simulink model "SIM_NARENDRA_4_METODO_DIFERENCIAL"  (R2012a)
settings: Solver=ode3  StartTime=0.0  StopTime=2.5  FixedStep=1e-4  RelTol=1e-3
libraries: simulink x1
settings Model: Creator=user  LastModifiedBy=user
settings DataIOCC: LimitDataPoints=on  SaveFormat=Array  ReturnWorkspaceOutputs=off
settings OptimizationCC: LifeSpan=inf  SimCompilerOptimization=Off
settings DebuggingCC: FcnCallInpInsideContextMsg=Enable All  SFUnexpectedBacktrackingDiag=warning  SFNoUnconditionalDefaultTransitionDiag=warning
settings HardwareCC: ProdBitPerPointer=32  ProdLargestAtomicFloat=None  ProdIntDivRoundTo=Undefined  ProdEndianess=Unspecified  ProdWordSize=32  ProdHWDeviceType=32-bit Generic
settings ModelReferenceCC: PropagateSignalLabelsOutOfModel=off
settings SFSimCC: SimUseLocalCustomCode=off
settings RTWCC: RTWUseLocalCustomCode=off  RTWCompilerOptimization=Off
settings GRTTargetCC: CodeReplacementLibrary=C89/C90 (ANSI)  GeneratePreprocessorConditionals=Disable all  CPPClassGenCompliant=off

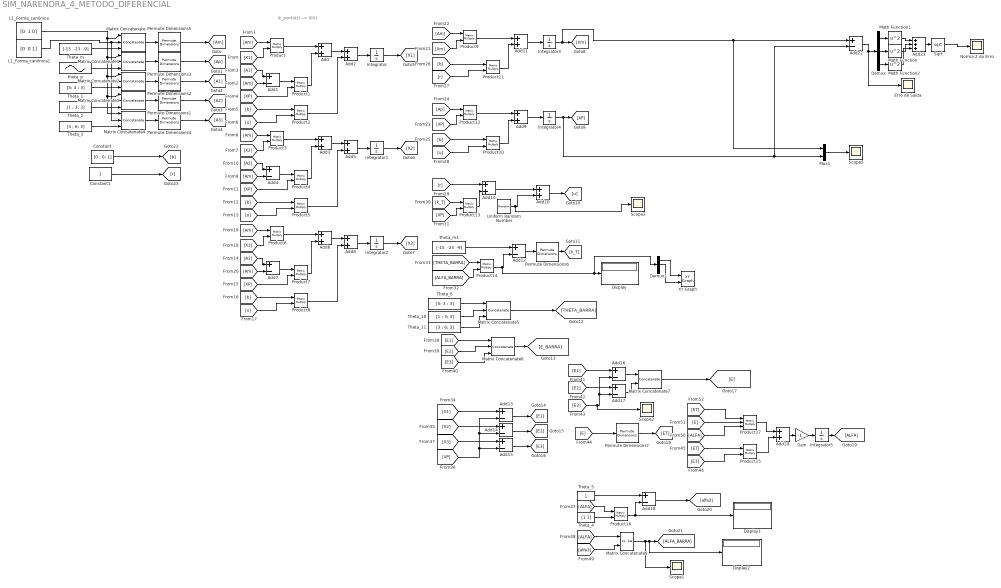
== system SIM_NARENDRA_4_METODO_DIFERENCIAL ==
  note: Xi_ponto(t) --> Xi(t)
  Add{,2..3,5..6,8..11,19..20} (11 alike) : Sum
  Add{1,4,7,12..18,22} (11 alike) : Sum  Inputs=+-
  Add23 : Sum  Inputs=+++
  Constant : Constant  Value=[0 ; 0; 1]
  Constant1 : Constant
  Demux : Demux  Outputs=3
  Demux1 : Demux  Outputs=3
  Display : Display
  Display2 : Display
  Display3 : Display
  Erro de Saída : Scope
      settings: SaveName=ScopeData6  YMin=-1.11044  YMax=1.99383
  Gain : Gain  Gain=-1
  Integrator : Integrator  InitialCondition=[2 2 1]
  Integrator1 : Integrator  InitialCondition=[1 0 2]
  Integrator2 : Integrator  InitialCondition=[0 0 1]
  Integrator3 : Integrator
  Integrator4 : Integrator  InitialCondition=[0.01 0.8 0.02]
  Integrator5 : Integrator
  L1_Forma_canônica : Constant  Value="[0  1 0]"
  L1_Forma_canônica1 : Constant  Value="[0  0 1]"
  Math Function : Math  Operator=square  SaturateOnIntegerOverflow=on
  Math Function1 : Math  Operator=square  SaturateOnIntegerOverflow=on
  Math Function2 : Math  Operator=square  SaturateOnIntegerOverflow=on
  Matrix Concatenate{,1..6} (7 alike) : Concatenate  NumInputs=3  Mode=Multidimensional array  ConcatenateDimension=2
  Matrix Concatenate7 : Concatenate  Mode=Multidimensional array  ConcatenateDimension=2
  Matrix Concatenate8 : Concatenate
  Mux1 : Mux  Inputs=2
  Norma 2 do Erro : Scope
      settings: SaveName=ScopeData5  YMin=-0.221046  YMax=1.99518
  Permute Dimensions{1..7} (7 alike) : PermuteDimensions
  Product{,1..16} (17 alike) : Product  Multiplication=Matrix(*)
  Product17 : Product  Inputs=3  Multiplication=Matrix(*)
  Scope{1..3,5} (4 alike) : Scope
      Scope1 settings: YMin=-2250  YMax=2500
      Scope2 settings: YMin=-0.5  YMax=5.5  SaveName=ScopeData2
      Scope3 settings: YMin=-1  YMax=1  SaveName=ScopeData3
      Scope5 settings: SaveName=ScopeData7  YMin=-1.90506  YMax=1.10057
  Sqrt : Sqrt  SaturateOnIntegerOverflow=on
  Theta_1 : Constant  Value=[5; 3 ; 3]
  Theta_10 : Constant  Value=[1 ; 3; 3]
  Theta_11 : Constant  Value=[3 ; 6; 3]
  Theta_2 : Constant  Value=[1 ; 3; 3]
  Theta_3 : Constant  Value=[3 ; 6; 3]
  Theta_4 : Constant  Value=[1 1]
  Theta_5 : Constant
  Theta_6 : Constant  Value=[5; 3 ; 3]
  Theta_m : Constant  Value="[-15  -23  -9]"
  Theta_m1 : Constant  Value="[-15  -23  -9]"
  Uniform Random Number : UniformRandomNumber
  XY Graph : simulink/Sinks/XY Graph  xmin=2  xmax=6  ymin=4  ymax=8  st=-1
  theta_p : Sin  Amplitude=[1 1 0]  Bias=[3 4 3]  Frequency=[1 1 0]  Phase=[pi/2 0 0]  SampleTime=0
  wires:
  Theta_m/1 -> Matrix Concatenate/3
  L1_Forma_canônica/1 -> Matrix Concatenate4/1, Matrix Concatenate3/1, Matrix Concatenate2/1, Matrix Concatenate1/1, Matrix Concatenate/1
  theta_p/1 -> Matrix Concatenate1/3
  Theta_1/1 -> Matrix Concatenate2/3
  Theta_2/1 -> Matrix Concatenate3/3
  Theta_3/1 -> Matrix Concatenate4/3
  Matrix Concatenate/1 -> Permute Dimensions5/1
  Matrix Concatenate1/1 -> Permute Dimensions3/1
  Matrix Concatenate2/1 -> Permute Dimensions2/1
  Matrix Concatenate3/1 -> Permute Dimensions1/1
  Matrix Concatenate4/1 -> Permute Dimensions4/1
  Permute Dimensions4/1 -> [A3]
  Permute Dimensions1/1 -> [A2]
  Permute Dimensions2/1 -> [A1]
  Permute Dimensions3/1 -> [Ap]
  Permute Dimensions5/1 -> [Am]
  [Am] -> Product/1
  [X1] -> Product/2
  Product/1 -> Add/1
  Product1/1 -> Add/2
  Add1/1 -> Product1/1
  [Am] -> Add1/2
  [A1] -> Add1/1
  [XP] -> Product1/2
  Add/1 -> Add2/1
  Product2/1 -> Add2/2
  [b] -> Product2/1
  [u] -> Product2/2
  Add2/1 -> Integrator/1
  Integrator/1 -> [X1]
  [Am] -> Product3/1
  [X2] -> Product3/2
  Product3/1 -> Add3/1
  Product4/1 -> Add3/2
  Add4/1 -> Product4/1
  [Am] -> Add4/2
  [A2] -> Add4/1
  [XP] -> Product4/2
  Add3/1 -> Add5/1
  Product5/1 -> Add5/2
  [b] -> Product5/1
  [u] -> Product5/2
  Add5/1 -> Integrator1/1
  Integrator1/1 -> [X2]
  [X3] -> Product6/2
  Product6/1 -> Add6/1
  Product7/1 -> Add6/2
  Add7/1 -> Product7/1
  [Am] -> Add7/2
  [A3] -> Add7/1
  [XP] -> Product7/2
  Add6/1 -> Add8/1
  Product8/1 -> Add8/2
  [b] -> Product8/1
  [u] -> Product8/2
  Add8/1 -> Integrator2/1
  Integrator2/1 -> [X3]
  [Am] -> Product6/1
  [Xm] -> Product9/2
  Product9/1 -> Add11/1
  Product11/1 -> Add11/2
  [b] -> Product11/1
  [r] -> Product11/2
  Add11/1 -> Integrator3/1
  [Am] -> Product9/1
  [XP] -> Product12/2
  Product12/1 -> Add9/1
  Product10/1 -> Add9/2
  [b] -> Product10/1
  [u] -> Product10/2
  Add9/1 -> Integrator4/1
  [Ap] -> Product12/1
  [k_T] -> Product13/1
  [XP] -> Product13/2
  Product13/1 -> Add10/2
  [r] -> Add10/1
  Permute Dimensions6/1 -> [k_T]
  [THETA_BARRA] -> Product14/1
  [ALFA_BARRA] -> Product14/2
  Theta_m1/1 -> Add12/1
  Product14/1 -> Demux1/1, Display/1, Add12/2
  Add12/1 -> Permute Dimensions6/1
  Theta_6/1 -> Matrix Concatenate5/1
  Theta_10/1 -> Matrix Concatenate5/2
  Theta_11/1 -> Matrix Concatenate5/3
  Matrix Concatenate5/1 -> [THETA_BARRA]
  [X1] -> Add13/1
  [XP] -> Add15/2, Add14/2, Add13/2
  [X2] -> Add14/1
  [X3] -> Add15/1
  Add13/1 -> [E1]
  Add14/1 -> [E2]
  Add15/1 -> [E3]
  Matrix Concatenate6/1 -> [E_BARRA]
  [E1] -> Matrix Concatenate6/1
  [E2] -> Matrix Concatenate6/2
  [E3] -> Matrix Concatenate6/3
  [E3] -> Scope2/1, Add17/2, Add16/2
  [E1] -> Add16/1
  [E2] -> Add17/1
  Add17/1 -> Matrix Concatenate7/2
  Add16/1 -> Matrix Concatenate7/1
  [E] -> Permute Dimensions7/1
  [ET] -> Product15/1
  [ALFA] -> Product16/1
  Theta_4/1 -> Product16/2
  Theta_5/1 -> Add18/1
  Product16/1 -> Display3/1, Add18/2
  [ALFA] -> Matrix Concatenate8/1
  [alfa3] -> Matrix Concatenate8/2
  Matrix Concatenate8/1 -> Scope1/1, Display2/1, [ALFA_BARRA]
  Constant/1 -> [b]
  Constant1/1 -> [r]
  Matrix Concatenate7/1 -> [E]
  Product15/1 -> Add19/2
  Add18/1 -> [alfa3]
  [E3] -> Product15/2
  Permute Dimensions7/1 -> [ET]
  [ALFA] -> Product17/3
  Product17/1 -> Add19/1
  Add19/1 -> Gain/1
  Integrator5/1 -> [ALFA]
  Gain/1 -> Integrator5/1
  [E] -> Product17/2
  [ET] -> Product17/1
  Add10/1 -> Add20/1
  Uniform Random Number/1 -> Scope3/1, Add20/2
  Add20/1 -> [u]
  L1_Forma_canônica1/1 -> Matrix Concatenate4/2, Matrix Concatenate3/2, Matrix Concatenate2/2, Matrix Concatenate1/2, Matrix Concatenate/2
  Integrator3/1 -> Mux1/1, Add22/1, [Xm]
  Integrator4/1 -> Add22/2, Mux1/2, [XP]
  Mux1/1 -> Scope5/1
  Sqrt/1 -> Norma 2 do Erro/1
  Add22/1 -> Erro de Saída/1, Demux/1
  Demux/2 -> Math Function/1
  Demux/1 -> Math Function1/1
  Math Function1/1 -> Add23/1
  Math Function/1 -> Add23/2
  Add23/1 -> Sqrt/1
  Demux/3 -> Math Function2/1
  Math Function2/1 -> Add23/3
  Demux1/1 -> XY Graph/1
  Demux1/2 -> XY Graph/2
